simulink model "Gerardo_IoT"  (R2018a)
settings: Solver=ode23  StartTime=0.0  StopTime=1.5  RelTol=1e-6  EnableMultiTasking=on
values from neighbouring files (symbols this model uses):
  Dir = value(4)    [interfaz.m]
  F = value(3)    [interfaz.m]
  Fc = value(2)    [interfaz.m]
  m = value(5)    [interfaz.m]
  Tm = value(7)    [interfaz.m]
  VL = value(6)    [interfaz.m]
undefined symbols (not defined in the file or in its folder): checker_board
libraries: powerlib x7, powerlib_meascontrol x4, visionsources x4
settings Model: Creator=LENOVO  LastModifiedBy=YAIR DURAN
settings DataIOCC: LimitDataPoints=on  SaveFormat=Array
settings OptimizationCC: LifeSpan=inf
settings DebuggingCC: SolverPrmCheckMsg=warning  SFUnexpectedBacktrackingDiag=warning  SFNoUnconditionalDefaultTransitionDiag=warning  SFExecutionAtInitializationDiag=none
settings HardwareCC: ProdBitPerPointer=32  ProdBitPerSizeT=32  ProdBitPerPtrDiffT=32  ProdLargestAtomicFloat=None  ProdIntDivRoundTo=Undefined  ProdEndianess=Unspecified  ProdWordSize=32  ProdHWDeviceType=32-bit Generic
settings ModelReferenceCC: PropagateSignalLabelsOutOfModel=off
settings CodeAppCC: StateflowObjectComments=on
settings GRTTargetCC: TargetLangStandard=C89/C90 (ANSI)  GeneratePreprocessorConditionals=Disable all
settings ConfigComp: CovMetricSettings=dw  CovHtmlReporting=on  CovSaveCumulativeToWorkspaceVar=on  CovSaveSingleToWorkspaceVar=on  CovExternalEMLEnable=off  CovSFcnEnable=off
settings SimscapeCC: SimscapeNormalizeSystem=off

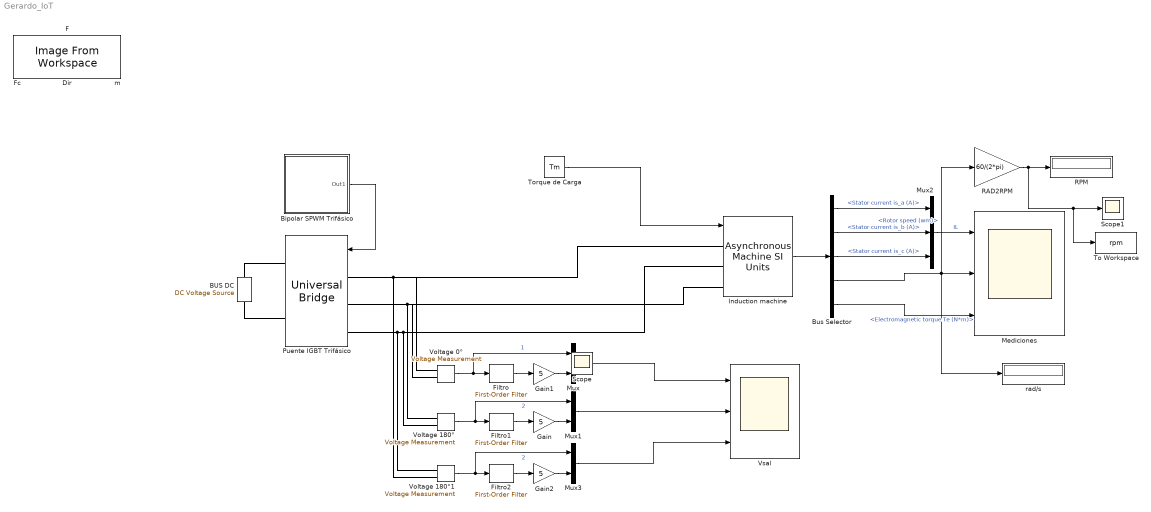
== system Gerardo_IoT ==
  BUS DC : powerlib/Electrical Sources/DC Voltage Source  Amplitude=sqrt(2)*VL*0.94  Measurements=None
  Bipolar SPWM Trifásico : Subsystem  mask{Fc=Fc, F=F, m=m, Dir=Dir}
      mask Display: plot([0 1 1 2 2 3 3 4 5 5 6 7 7 8 9 10 11 12 12 13 14 14 15 16 16 17 17 18 18 19],[0 0 1 1 0 0 1 1 1 0 0 0 1 1 1 1 1 1 0 0 0 1 1 1 0 0 1 1 0 0])
  Bus Selector : BusSelector  OutputSignals=Stator measurements.Stator current is_a (A),Stator measurements.Stator current is_b (A),Stator measurements.Stator current is_c (A),Mechanical.Rotor speed (wm),Mechanical.Electromagnetic torque Te (N*m)
  Filtro : powerlib_meascontrol/Filters/First-Order Filter  FilterType=Lowpass  Tc=0.02  Ts=0  Initialize=on  Vac_Init=[1, 0, F ]  Vdc_Init=0  PlotResponse=off  FreqRange="[0,  200,  1]"
      settings: SourceProductName=Simscape Power Systems
  Filtro1 : powerlib_meascontrol/Filters/First-Order Filter  FilterType=Lowpass  Tc=0.02  Ts=0  Initialize=on  Vac_Init=[1, 0, F]  Vdc_Init=0  PlotResponse=off  FreqRange="[0,  200,  1]"
      settings: SourceProductName=Simscape Power Systems
  Filtro2 : powerlib_meascontrol/Filters/First-Order Filter  FilterType=Lowpass  Tc=0.02  Ts=0  Initialize=on  Vac_Init=[1, 0, F]  Vdc_Init=0  PlotResponse=off  FreqRange="[0,  200,  1]"
      settings: SourceProductName=Simscape Power Systems
  Gain : Gain  Gain=5
  Gain1 : Gain  Gain=5
  Gain2 : Gain  Gain=5
  Induction machine : powerlib/Machines/Asynchronous Machine SI Units  RotorType=Squirrel-cage  PresetModel=No  MechanicalLoad=Torque Tm  ShowDetailedParameters=on  ReferenceFrame=Stationary  Units=SI  MeasurementBus=off  NominalParameters=[2238,220,60]  Stator=[0.435,0.002]  Rotor=[0.816,0.002]  Cage1=[ 0.022 0.226/377]  Cage2=[ 0.022 0.226/377]  Lm=69.31e-3  Mechanical=[0.089,0.005,2]  PolePairs=2  InitialConditions=[1,0,0,0,0,0,0,0]  SimulateSaturation=off  Saturation=[0 0;0 0]  LoadFlowParameters=0  TsPowergui=0  TsBlock=-1  IterativeModel=Forward Euler  IterativeDiscreteModel=Trapezoidal non iterative  Pmec=0
  "Mediciones " : Scope  NumInputPorts=3
  Mux : Mux  Inputs=2
  Mux1 : Mux  Inputs=2
  Mux2 : Mux  Inputs=3
  Mux3 : Mux  Inputs=2
  Puente IGBT Trifásico : powerlib/Power Electronics/Universal Bridge  Arms=3  SnubberResistance=1e5  SnubberCapacitance=inf  Device=IGBT / Diodes  Ron=1e-3  Lon=0  ForwardVoltages="[  0  0  ]"  ForwardVoltage=0  GTOparameters=[ 10e-6 , 20e-6 ]  IGBTparameters=[ 1e-6 , 2e-6 ]  Measurements=None  Measurements_2=None  converterType=Rectifier
  RAD2RPM : Gain  Gain=60/(2*pi)  RndMeth=Round
  RPM : Display
  Scope : Scope
  Scope1 : Scope
  To Workspace : ToWorkspace  VariableName=rpm  SampleTime=-1
      settings: MaxDataPoints=1  Save2DSignal=2-D array (concatenate along first dimension)
  Torque de Carga : Constant  Value=Tm
  Voltage 0° : powerlib/Measurements/Voltage Measurement  PhasorSimulation=off  OutputType=Complex  PSBequivalent=0
  Voltage 180° : powerlib/Measurements/Voltage Measurement  PhasorSimulation=off  OutputType=Complex  PSBequivalent=0
  Voltage 180°1 : powerlib/Measurements/Voltage Measurement  PhasorSimulation=off  OutputType=Complex  PSBequivalent=0
  Vsal : Scope  NumInputPorts=3
  rad/s : Display
  Dir : visionsources/Image From Workspace  Tag=vipblks_nd  IOType=siggen  ImageValue=checker_board(10)  Ts=inf  imagePorts=One multidimensional signal  OutPortLabels=R|G|B  ImageDataType=Inherit from 'Value'  Signed=on  WordLength=16  sdImageDataType=sfix(16)  FractionLengthMode=User-defined  FractionLength=15
      settings: SourceProductName=Computer Vision System Toolbox  SourceProductBaseCode=VP
  F : visionsources/Image From Workspace  Tag=vipblks_nd  IOType=siggen  ImageValue=checker_board(10)  Ts=inf  imagePorts=One multidimensional signal  OutPortLabels=R|G|B  ImageDataType=Inherit from 'Value'  Signed=on  WordLength=16  sdImageDataType=sfix(16)  FractionLengthMode=User-defined  FractionLength=15
      settings: SourceProductName=Computer Vision System Toolbox  SourceProductBaseCode=VP
  Fc : visionsources/Image From Workspace  Tag=vipblks_nd  IOType=siggen  ImageValue=checker_board(10)  Ts=inf  imagePorts=One multidimensional signal  OutPortLabels=R|G|B  ImageDataType=Inherit from 'Value'  Signed=on  WordLength=16  sdImageDataType=sfix(16)  FractionLengthMode=User-defined  FractionLength=15
      settings: SourceProductName=Computer Vision System Toolbox  SourceProductBaseCode=VP
  m : visionsources/Image From Workspace  Tag=vipblks_nd  IOType=siggen  ImageValue=checker_board(10)  Ts=inf  imagePorts=One multidimensional signal  OutPortLabels=R|G|B  ImageDataType=Inherit from 'Value'  Signed=on  WordLength=16  sdImageDataType=sfix(16)  FractionLengthMode=User-defined  FractionLength=15
      settings: SourceProductName=Computer Vision System Toolbox  SourceProductBaseCode=VP
  wires:
  Bipolar SPWM Trifásico/1(Out1) -> Puente IGBT Trifásico/1
  Voltage 0°/1 -> Mux/1, Filtro/1  "1"
  Voltage 180°/1 -> Mux1/1, Filtro1/1  "2"
  Filtro1/1 -> Gain/1
  Gain/1 -> Mux1/2
  Filtro/1 -> Gain1/1
  Gain1/1 -> Mux/2
  Torque de Carga/1 -> Induction machine/1
  Voltage 180°1/1 -> Filtro2/1, Mux3/1  "2"
  Filtro2/1 -> Gain2/1
  Gain2/1 -> Mux3/2
  Mux/1 -> Vsal/1
  Mux1/1 -> Vsal/2
  Mux3/1 -> Vsal/3
  Induction machine/1 -> Bus Selector/1
  Bus Selector/1 -> Mux2/1  "<Stator current is_a (A)>"
  Bus Selector/2 -> Mux2/2  "<Stator current is_b (A)>"
  Bus Selector/3 -> Mux2/3  "<Stator current is_c (A)>"
  Mux2/1 -> "Mediciones "/1  "IL"
  Bus Selector/4 -> rad/s/1, RAD2RPM/1, "Mediciones "/2  "<Rotor speed (wm)>"
  Bus Selector/5 -> "Mediciones "/3  "<Electromagnetic torque Te (N*m)>"
  RAD2RPM/1 -> To Workspace/1, Scope1/1, RPM/1
  connections:
  Puente IGBT Trifásico/RConn1 -- BUS DC/RConn1
  Puente IGBT Trifásico/RConn2 -- BUS DC/LConn1
  Induction machine/LConn1 -- Voltage 0°/LConn1 -- Voltage 180°1/LConn2 -- Puente IGBT Trifásico/LConn1
  Puente IGBT Trifásico/LConn2 -- Induction machine/LConn3 -- Voltage 0°/LConn2 -- Voltage 180°/LConn1
  Voltage 180°/LConn2 -- Induction machine/LConn2 -- Voltage 180°1/LConn1 -- Puente IGBT Trifásico/LConn3

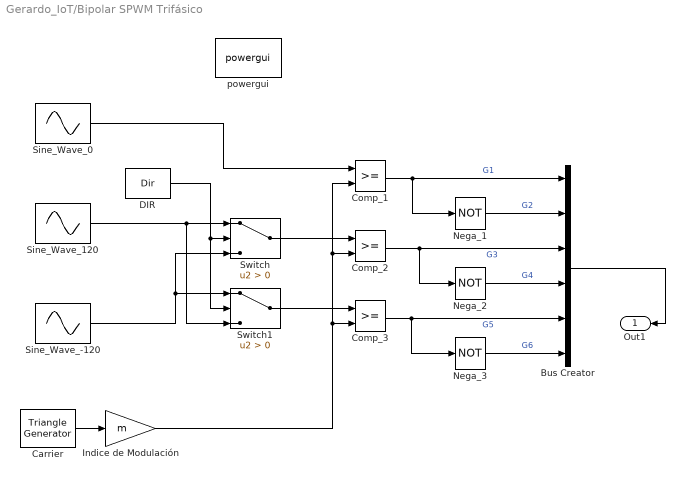
== system Gerardo_IoT/Bipolar SPWM Trifásico ==
  Bus Creator : BusCreator  Inputs=6
  Carrier : powerlib_meascontrol/Pulse & Signal Generators/Triangle Generator  Freq=Fc  Phase=0  Ts=0
  Comp_1 : RelationalOperator  OutDataTypeStr=boolean  RndMeth=Nearest
  Comp_2 : RelationalOperator  OutDataTypeStr=boolean  RndMeth=Nearest
  Comp_3 : RelationalOperator  OutDataTypeStr=boolean  RndMeth=Nearest
  DIR : Constant  Value=Dir
  Indice de Modulación : Gain  Gain=m
  Nega_1 : Logic  Operator=NOT  AllPortsSameDT=off  OutDataTypeStr=boolean
  Nega_2 : Logic  Operator=NOT  AllPortsSameDT=off  OutDataTypeStr=boolean
  Nega_3 : Logic  Operator=NOT  AllPortsSameDT=off  OutDataTypeStr=boolean
  Sine_Wave_-120 : Sin  Frequency=2*pi*F  Phase=-2*pi/3  SampleTime=0
  Sine_Wave_0 : Sin  Frequency=2*pi*F  SampleTime=0
  Sine_Wave_120 : Sin  Frequency=2*pi*F  Phase=2*pi/3  SampleTime=0
  Switch : Switch  Criteria=u2 > Threshold
  Switch1 : Switch  Criteria=u2 > Threshold
  powergui : powerlib/powergui  Priority=1  SimulationMode=Discrete  SampleTime=50e-6  frequency=60  Iterations=50  frequencyindice=0  Pbase=100e6  ErrMax=1e-4  UnitsV=kV  UnitsW=MW  buscounter=0  FunctionMessages=off  echomessages=off  EnableUseOfTLC=off  CurrentSourceSwitches=off  DisableSnubberDevices=off  DisableRonSwitches=off  DisableVfSwitches=off  DisplayEquations=off  SolverType=Tustin  Interpol=off  ExternalGateDelay=off  methode=off  Ts=0  x0status=blocks  SPID=off  SwTol=0  HookPort=off  RestoreLinks=warning  ResistiveCurrentMeasurement=off  Frange=[0:2:500]  Ylog=off  Xlog=on  ShowGrid=off  save=off  variable=ZData  structure=0  ZoomFFT=off  StartTime=0.0  cycles=1  DisplayStyle=1  fundamental=60  FreqAxis=off  MaxFrequency=1000  frequencyindicesteady=1  RmsSteady=1  display=off
  Out1 : Outport
  wires:
  Sine_Wave_0/1 -> Comp_1/1
  Nega_2/1 -> Bus Creator/4  "G4"
  Nega_1/1 -> Bus Creator/2  "G2"
  Comp_2/1 -> Bus Creator/3, Nega_2/1  "G3"
  Comp_3/1 -> Bus Creator/5, Nega_3/1  "G5"
  Nega_3/1 -> Bus Creator/6  "G6"
  Comp_1/1 -> Bus Creator/1, Nega_1/1  "G1"
  Bus Creator/1 -> Out1/1
  Carrier/1 -> Indice de Modulación/1
  Indice de Modulación/1 -> Comp_1/2, Comp_2/2, Comp_3/2
  Sine_Wave_120/1 -> Switch1/3, Switch/1
  Sine_Wave_-120/1 -> Switch/3, Switch1/1
  Switch/1 -> Comp_2/1
  Switch1/1 -> Comp_3/1
  DIR/1 -> Switch1/2, Switch/2
